simulink model "airTrackInelastic"  (R2021a)
settings: Solver=VariableStepAuto  StartTime=0.0  StopTime=30  FixedStep=0.02  MaxStep=0.01  RelTol=1e-6  EnableMultiTasking=on
PostLoadFcn:
  | disp('default settings')
  | 
  | % Default starting positions
  | x0_cart1 = -0.2
  | x0_cart2 = 0.8
  | x0_gate1 = -0.4
  | x0_gate2 = 0.4
  | 
  | % How much damping the carts feel
  | dampingCoef = 0.01 % N/(m/s)
  | 
  | % Max measurement noise for the gates
  | noise_max = 0.01 % seconds
  | 
  | % How many time steps to show in the history
  | nHistory = 4
  | 
  | % Based on the provided STLs
  | cart_length = 0.15
  | 
  | subsystems = find_system(gcs,'BlockType','SubSystem');
  | p = Simulink.Mask.get(subsystems{1});
  | p.Parameters(1).Value = '-0.8';
  | p.Parameters(2).Value = '0';
  | p.Parameters(3).Value = '-0.4';
  | p.Parameters(4).Value = '0.4';
  | p.Parameters(5).Value = '0';
  | p.Parameters(6).Value = '0';
undefined symbols (not defined in the file): Push, X, x, Y, Z
libraries: sm_lib x54, simulink x12, nesl_utility x11
(part 2 of 2)

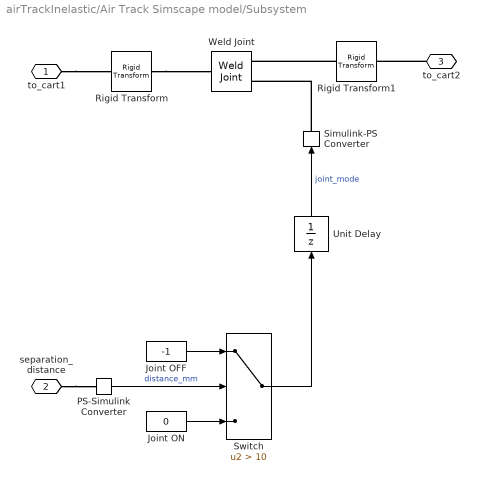
== system airTrackInelastic/Air Track Simscape model/Subsystem ==
  Joint OFF : Constant  Value=-1
  Joint ON : Constant  Value=0
  PS-Simulink Converter : nesl_utility/PS-Simulink Converter  PhysicalDomain=network_engine_domain  SubClassName=ps_output  LeftPortType=input  RightPortType=output  PseudoPeriodic=off  Frequencies=[]  Unit=mm  AffineConversion=off
      settings: SourceProductBaseCode=PW,SS
  Rigid Transform : sm_lib/Frames and Transforms/Rigid Transform  TranslationMethod=StandardAxis  TranslationStandardOffset=-0.0075  TranslationLengthUnit=m  TranslationStandardAxis=+X  TranslationCartesianOffset=[0 0 0]  TranslationROffset=0  TranslationROffsetUnits=m  TranslationZOffset=0  TranslationZOffsetUnits=m  TranslationThetaOffset=0  TranslationThetaOffsetUnits=deg  RotationMethod=None  RotationAngleUnits=deg  RotationStandardAxis=+Z  RotationAngle=0.0  RotationArbitraryAxis=[0 0 1]  FollAlignAxisA=+X  BaseAlignAxisA=+Y  FollAlignAxisB=+Y  BaseAlignAxisB=+Z  RotationSequenceAxes=FollowerAxes  RotationSequence=XYX  RotationSequenceAngles=[0 0 0]  RotationSequenceAnglesUnits=deg  RotationMatrix=[1 0 0; 0 1 0; 0 0 1]
  Rigid Transform1 : sm_lib/Frames and Transforms/Rigid Transform  TranslationMethod=StandardAxis  TranslationStandardOffset=0.0075  TranslationLengthUnit=m  TranslationStandardAxis=-X  TranslationCartesianOffset=[0 0 0]  TranslationROffset=0  TranslationROffsetUnits=m  TranslationZOffset=0  TranslationZOffsetUnits=m  TranslationThetaOffset=0  TranslationThetaOffsetUnits=deg  RotationMethod=None  RotationAngleUnits=deg  RotationStandardAxis=+Z  RotationAngle=0.0  RotationArbitraryAxis=[0 0 1]  FollAlignAxisA=+X  BaseAlignAxisA=+Y  FollAlignAxisB=+Y  BaseAlignAxisB=+Z  RotationSequenceAxes=FollowerAxes  RotationSequence=XYX  RotationSequenceAngles=[0 0 0]  RotationSequenceAnglesUnits=deg  RotationMatrix=[1 0 0; 0 1 0; 0 0 1]
  Simulink-PS Converter : nesl_utility/Simulink-PS Converter  PhysicalDomain=network_engine_domain  SubClassName=ps_input  LeftPortType=input  RightPortType=output  PseudoPeriodic=off  Frequencies=[]  NoiseDistribution=none  NoiseParameters=[]  Unit=1  AffineConversion=off  FilteringAndDerivatives=provide  SimscapeFilterOrder=1  InputFilterTimeConstant=0.001  UdotUserProvided=0
      settings: SourceProductBaseCode=PW,SS
  Switch : Switch  Criteria=u2 > Threshold  Threshold=10
  Unit Delay : UnitDelay  InitialCondition=-1  SampleTime=0.01  HasFrameUpgradeWarning=on
  Weld Joint : sm_lib/Joints/Weld Joint  JointMode=ProvidedByInput  SenseConstraintForce=off  SenseConstraintForceX=off  SenseConstraintForceY=off  SenseConstraintForceZ=off  SenseConstraintTorque=off  SenseConstraintTorqueX=off  SenseConstraintTorqueY=off  SenseConstraintTorqueZ=off  SenseTotalForce=off  SenseTotalForceX=off  SenseTotalForceY=off  SenseTotalForceZ=off  SenseTotalTorque=off  SenseTotalTorqueX=off  SenseTotalTorqueY=off  SenseTotalTorqueZ=off  CompositeWrenchDir=FollowerOnBase  CompositeWrenchFrame=BaseFrame
  to_cart1 : PMIOPort  Side=Left
  separation_distance : PMIOPort  Port=2  Side=Left
  to_cart2 : PMIOPort  Port=3  Side=Right
  wires:
  PS-Simulink Converter/1 -> Switch/2  "distance_mm"
  Joint OFF/1 -> Switch/1
  Joint ON/1 -> Switch/3
  Unit Delay/1 -> Simulink-PS Converter/1  "joint_mode"
  Switch/1 -> Unit Delay/1
  connections:
  to_cart2/RConn1 -- Rigid Transform1/RConn1
  Simulink-PS Converter/RConn1 -- Weld Joint/LConn2
  to_cart1/RConn1 -- Rigid Transform/LConn1
  separation_distance/RConn1 -- PS-Simulink Converter/LConn1
  Rigid Transform/RConn1 -- Weld Joint/RConn1
  Rigid Transform1/LConn1 -- Weld Joint/LConn1

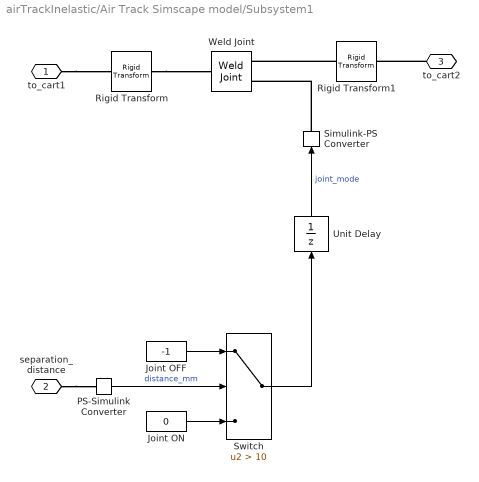
== system airTrackInelastic/Air Track Simscape model/Subsystem1 ==
  Joint OFF : Constant  Value=-1
  Joint ON : Constant  Value=0
  PS-Simulink Converter : nesl_utility/PS-Simulink Converter  PhysicalDomain=network_engine_domain  SubClassName=ps_output  LeftPortType=input  RightPortType=output  PseudoPeriodic=off  Frequencies=[]  Unit=mm  AffineConversion=off
      settings: SourceProductBaseCode=PW,SS
  Rigid Transform : sm_lib/Frames and Transforms/Rigid Transform  TranslationMethod=StandardAxis  TranslationStandardOffset=-0.0075  TranslationLengthUnit=m  TranslationStandardAxis=+X  TranslationCartesianOffset=[0 0 0]  TranslationROffset=0  TranslationROffsetUnits=m  TranslationZOffset=0  TranslationZOffsetUnits=m  TranslationThetaOffset=0  TranslationThetaOffsetUnits=deg  RotationMethod=None  RotationAngleUnits=deg  RotationStandardAxis=+Z  RotationAngle=0.0  RotationArbitraryAxis=[0 0 1]  FollAlignAxisA=+X  BaseAlignAxisA=+Y  FollAlignAxisB=+Y  BaseAlignAxisB=+Z  RotationSequenceAxes=FollowerAxes  RotationSequence=XYX  RotationSequenceAngles=[0 0 0]  RotationSequenceAnglesUnits=deg  RotationMatrix=[1 0 0; 0 1 0; 0 0 1]
  Rigid Transform1 : sm_lib/Frames and Transforms/Rigid Transform  TranslationMethod=StandardAxis  TranslationStandardOffset=0.0075  TranslationLengthUnit=m  TranslationStandardAxis=-X  TranslationCartesianOffset=[0 0 0]  TranslationROffset=0  TranslationROffsetUnits=m  TranslationZOffset=0  TranslationZOffsetUnits=m  TranslationThetaOffset=0  TranslationThetaOffsetUnits=deg  RotationMethod=None  RotationAngleUnits=deg  RotationStandardAxis=+Z  RotationAngle=0.0  RotationArbitraryAxis=[0 0 1]  FollAlignAxisA=+X  BaseAlignAxisA=+Y  FollAlignAxisB=+Y  BaseAlignAxisB=+Z  RotationSequenceAxes=FollowerAxes  RotationSequence=XYX  RotationSequenceAngles=[0 0 0]  RotationSequenceAnglesUnits=deg  RotationMatrix=[1 0 0; 0 1 0; 0 0 1]
  Simulink-PS Converter : nesl_utility/Simulink-PS Converter  PhysicalDomain=network_engine_domain  SubClassName=ps_input  LeftPortType=input  RightPortType=output  PseudoPeriodic=off  Frequencies=[]  NoiseDistribution=none  NoiseParameters=[]  Unit=1  AffineConversion=off  FilteringAndDerivatives=provide  SimscapeFilterOrder=1  InputFilterTimeConstant=0.001  UdotUserProvided=0
      settings: SourceProductBaseCode=PW,SS
  Switch : Switch  Criteria=u2 > Threshold  Threshold=10
  Unit Delay : UnitDelay  InitialCondition=-1  SampleTime=0.01  HasFrameUpgradeWarning=on
  Weld Joint : sm_lib/Joints/Weld Joint  JointMode=ProvidedByInput  SenseConstraintForce=off  SenseConstraintForceX=off  SenseConstraintForceY=off  SenseConstraintForceZ=off  SenseConstraintTorque=off  SenseConstraintTorqueX=off  SenseConstraintTorqueY=off  SenseConstraintTorqueZ=off  SenseTotalForce=off  SenseTotalForceX=off  SenseTotalForceY=off  SenseTotalForceZ=off  SenseTotalTorque=off  SenseTotalTorqueX=off  SenseTotalTorqueY=off  SenseTotalTorqueZ=off  CompositeWrenchDir=FollowerOnBase  CompositeWrenchFrame=BaseFrame
  to_cart1 : PMIOPort  Side=Left
  separation_distance : PMIOPort  Port=2  Side=Left
  to_cart2 : PMIOPort  Port=3  Side=Right
  wires:
  PS-Simulink Converter/1 -> Switch/2  "distance_mm"
  Joint OFF/1 -> Switch/1
  Joint ON/1 -> Switch/3
  Unit Delay/1 -> Simulink-PS Converter/1  "joint_mode"
  Switch/1 -> Unit Delay/1
  connections:
  to_cart2/RConn1 -- Rigid Transform1/RConn1
  Simulink-PS Converter/RConn1 -- Weld Joint/LConn2
  to_cart1/RConn1 -- Rigid Transform/LConn1
  separation_distance/RConn1 -- PS-Simulink Converter/LConn1
  Rigid Transform/RConn1 -- Weld Joint/RConn1
  Rigid Transform1/LConn1 -- Weld Joint/LConn1

== system airTrackInelastic/Air Track Simscape model/gate1 ==
  Constant : Constant  Value=x0_gate1
  Display : Display
  File Solid4 : sm_lib/Body Elements/File Solid  ExtGeomFileName=./stls/gate.stl  UnitType=Custom  ExtGeomFileUnits=mm  StepReaderType=HEX  ExportConvexHullGeometry=off  InertiaType=PointMass  Mass=180  MassUnits=g  CenterOfMass=[0 0 0]  CenterOfMassUnits=m  MomentsOfInertia=[1 1 1]  MomentsOfInertiaUnits=kg*m^2  ProductsOfInertia=[0 0 0]  ProductsOfInertiaUnits=kg*m^2  BasedOnType=Density  Density=1000  DensityUnits=kg/m^3  DoExposeReferenceFrame=on  SerializedFrames=<Frames><Frame><Id>Frame1</Id><Value><Name>F1</Name><Origin><Source>CenterOfMassFrame</Source><FeatureName></FeatureName></Origin><PrimaryAxis><DefinedDirection>+X</DefinedDirection><Source>ReferenceFrame</Source><SourceDirection>+Z</SourceDirection><FeatureName></FeatureName></PrimaryAxis><SecondaryAxis><DefinedDirection>+Y</DefinedDirection><Source>ReferenceFrame</Source><SourceDirection>+X</SourceDirection><FeatureName></FeatureName></SecondaryAxis></Value></Frame></Frames>  GraphicType=FromGeometry  MarkerShape=Sphere  MarkerSize=10  GraphicVisPropType=AdvancedVisualProperties  GraphicDiffuseColor="[0.8500    0.3250    0.0980]"  GraphicSpecularColor="[0.8    0.8   0.8 1]"  GraphicAmbientColor=[0.05 0.05 0.05 1]  GraphicEmissiveColor=[0.0 0.0 0.0 1.0]  GraphicShininess=50  GraphicOpacity=1.0
  Gate timing and history : Subsystem
  Rigid Transform : sm_lib/Frames and Transforms/Rigid Transform  TranslationMethod=Cartesian  TranslationStandardOffset=x0_cart2  TranslationLengthUnit=m  TranslationStandardAxis=+X  TranslationCartesianOffset=[-x0_gate1 0 0 ]  TranslationROffset=0  TranslationROffsetUnits=m  TranslationZOffset=0  TranslationZOffsetUnits=m  TranslationThetaOffset=0  TranslationThetaOffsetUnits=deg  RotationMethod=None  RotationAngleUnits=deg  RotationStandardAxis=+Z  RotationAngle=0.0  RotationArbitraryAxis=[0 0 1]  FollAlignAxisA=+X  BaseAlignAxisA=+Y  FollAlignAxisB=+Y  BaseAlignAxisB=+Z  RotationSequenceAxes=FollowerAxes  RotationSequence=XYX  RotationSequenceAngles=[0 0 0]  RotationSequenceAnglesUnits=deg  RotationMatrix=[1 0 0; 0 1 0; 0 0 1]
  File Solid3 : PMIOPort  Side=Right
  wires:
  Gate timing and history/1(Out1) -> Display/1
  Constant/1 -> Gate timing and history/1(gate_pos)
  connections:
  Rigid Transform/LConn1 -- File Solid3/RConn1
  File Solid4/RConn1 -- Rigid Transform/RConn1

== system airTrackInelastic/Air Track Simscape model/gate2 ==
  note: The cart has a mass of 180 grams and a length of 15cm
  Constant : Constant  Value=x0_gate2
  Display : Display
  File Solid4 : sm_lib/Body Elements/File Solid  ExtGeomFileName=./stls/gate.stl  UnitType=Custom  ExtGeomFileUnits=mm  StepReaderType=HEX  ExportConvexHullGeometry=off  InertiaType=PointMass  Mass=180  MassUnits=g  CenterOfMass=[0 0 0]  CenterOfMassUnits=m  MomentsOfInertia=[1 1 1]  MomentsOfInertiaUnits=kg*m^2  ProductsOfInertia=[0 0 0]  ProductsOfInertiaUnits=kg*m^2  BasedOnType=Density  Density=1000  DensityUnits=kg/m^3  DoExposeReferenceFrame=on  SerializedFrames=<Frames><Frame><Id>Frame1</Id><Value><Name>F1</Name><Origin><Source>CenterOfMassFrame</Source><FeatureName></FeatureName></Origin><PrimaryAxis><DefinedDirection>+X</DefinedDirection><Source>ReferenceFrame</Source><SourceDirection>+Z</SourceDirection><FeatureName></FeatureName></PrimaryAxis><SecondaryAxis><DefinedDirection>+Y</DefinedDirection><Source>ReferenceFrame</Source><SourceDirection>+X</SourceDirection><FeatureName></FeatureName></SecondaryAxis></Value></Frame></Frames>  GraphicType=FromGeometry  MarkerShape=Sphere  MarkerSize=10  GraphicVisPropType=AdvancedVisualProperties  GraphicDiffuseColor="[           0    0.4470    0.7410]"  GraphicSpecularColor="[0.8    0.8   0.8 1]"  GraphicAmbientColor=[0.05 0.05 0.05 1]  GraphicEmissiveColor=[0.0 0.0 0.0 1.0]  GraphicShininess=50  GraphicOpacity=1.0
  Gate timing and history : Subsystem
  Rigid Transform : sm_lib/Frames and Transforms/Rigid Transform  TranslationMethod=Cartesian  TranslationStandardOffset=x0_cart2  TranslationLengthUnit=m  TranslationStandardAxis=+X  TranslationCartesianOffset=[-x0_gate2 0 0]  TranslationROffset=0  TranslationROffsetUnits=m  TranslationZOffset=0  TranslationZOffsetUnits=m  TranslationThetaOffset=0  TranslationThetaOffsetUnits=deg  RotationMethod=None  RotationAngleUnits=deg  RotationStandardAxis=+Z  RotationAngle=0.0  RotationArbitraryAxis=[0 0 1]  FollAlignAxisA=+X  BaseAlignAxisA=+Y  FollAlignAxisB=+Y  BaseAlignAxisB=+Z  RotationSequenceAxes=FollowerAxes  RotationSequence=XYX  RotationSequenceAngles=[0 0 0]  RotationSequenceAnglesUnits=deg  RotationMatrix=[1 0 0; 0 1 0; 0 0 1]
  File Solid3 : PMIOPort  Side=Right
  wires:
  Constant/1 -> Gate timing and history/1(gate_pos)
  Gate timing and history/1(Out1) -> Display/1
  connections:
  File Solid4/RConn1 -- Rigid Transform/RConn1
  Rigid Transform/LConn1 -- File Solid3/RConn1

== system airTrackInelastic/Air Track Simscape model/stop1 ==
  File Solid2 : sm_lib/Body Elements/File Solid  ExtGeomFileName=./stls/stop.stl  UnitType=Custom  ExtGeomFileUnits=mm  StepReaderType=HEX  ExportConvexHullGeometry=off  InertiaType=PointMass  Mass=180  MassUnits=g  CenterOfMass=[0 0 0]  CenterOfMassUnits=m  MomentsOfInertia=[1 1 1]  MomentsOfInertiaUnits=kg*m^2  ProductsOfInertia=[0 0 0]  ProductsOfInertiaUnits=kg*m^2  BasedOnType=Density  Density=1000  DensityUnits=kg/m^3  DoExposeReferenceFrame=on  SerializedFrames=<Frames><Frame><Id>Frame1</Id><Value><Name>F1</Name><Origin><Source>CenterOfMassFrame</Source><FeatureName></FeatureName></Origin><PrimaryAxis><DefinedDirection>+X</DefinedDirection><Source>ReferenceFrame</Source><SourceDirection>+Z</SourceDirection><FeatureName></FeatureName></PrimaryAxis><SecondaryAxis><DefinedDirection>+Y</DefinedDirection><Source>ReferenceFrame</Source><SourceDirection>+X</SourceDirection><FeatureName></FeatureName></SecondaryAxis></Value></Frame></Frames>  GraphicType=FromGeometry  MarkerShape=Sphere  MarkerSize=10  GraphicVisPropType=AdvancedVisualProperties  GraphicDiffuseColor="[0.2   0.2    0.2]"  GraphicSpecularColor="[0.8    0.8   0.8 1]"  GraphicAmbientColor=[0.05 0.05 0.05 1]  GraphicEmissiveColor=[0.0 0.0 0.0 1.0]  GraphicShininess=50  GraphicOpacity=1.0
  Rigid Transform : sm_lib/Frames and Transforms/Rigid Transform  TranslationMethod=Cartesian  TranslationStandardOffset=0  TranslationLengthUnit=m  TranslationStandardAxis=+X  TranslationCartesianOffset=[0 0 0]  TranslationROffset=0  TranslationROffsetUnits=m  TranslationZOffset=0  TranslationZOffsetUnits=m  TranslationThetaOffset=0  TranslationThetaOffsetUnits=deg  RotationMethod=None  RotationAngleUnits=deg  RotationStandardAxis=+Z  RotationAngle=0.0  RotationArbitraryAxis=[0 0 1]  FollAlignAxisA=+X  BaseAlignAxisA=+Y  FollAlignAxisB=+Y  BaseAlignAxisB=+Z  RotationSequenceAxes=FollowerAxes  RotationSequence=XYX  RotationSequenceAngles=[0 0 0]  RotationSequenceAnglesUnits=deg  RotationMatrix=[1 0 0; 0 1 0; 0 0 1]
  Rigid Transform1 : sm_lib/Frames and Transforms/Rigid Transform  TranslationMethod=Cartesian  TranslationStandardOffset=1  TranslationLengthUnit=m  TranslationStandardAxis=+X  TranslationCartesianOffset=[1-0.012 -0.225 0]  TranslationROffset=0  TranslationROffsetUnits=m  TranslationZOffset=0  TranslationZOffsetUnits=m  TranslationThetaOffset=0  TranslationThetaOffsetUnits=deg  RotationMethod=None  RotationAngleUnits=deg  RotationStandardAxis=+Z  RotationAngle=0.0  RotationArbitraryAxis=[0 0 1]  FollAlignAxisA=+X  BaseAlignAxisA=+Y  FollAlignAxisB=+Y  BaseAlignAxisB=+Z  RotationSequenceAxes=FollowerAxes  RotationSequence=XYX  RotationSequenceAngles=[0 0 0]  RotationSequenceAnglesUnits=deg  RotationMatrix=[1 0 0; 0 1 0; 0 0 1]
  contact_ball1 : sm_lib/Body Elements/Spherical Solid  GraphicAmbientColor=[0.15 0.15 0.15 1.0]  BasedOnType=Density  CenterOfMass=[0 0 0]  CenterOfMassUnits=m  GraphicDiffuseColor="[ 0.9290    0.6940    0.1250]"  Density=1000  DensityUnits=kg/m^3  DoExposeReferenceFrame=on  GraphicEmissiveColor=[0.0 0.0 0.0 1.0]  ExportEntireGeometry=on  SerializedExposedGeometries=<ExposedGeometries><ExposedGeometry><RawGeometryId>entire</RawGeometryId><ExposedGeometryId>G</ExposedGeometryId></ExposedGeometry></ExposedGeometries>  SerializedFrames=<Frames/>  MarkerShape=Sphere  MarkerSize=10  GraphicType=FromGeometry  InertiaType=CalculateFromGeometry  Mass=1  MassUnits=kg  MomentsOfInertia=[1 1 1]  MomentsOfInertiaUnits=kg*m^2  GraphicOpacity=1.0  ProductsOfInertia=[0 0 0]  ProductsOfInertiaUnits=kg*m^2  GraphicShininess=75  GraphicSpecularColor=[0.5 0.5 0.5 1.0]  SphereRadius=0.0075  SphereRadiusUnits=m  GraphicVisPropType=SimpleVisualProperties
  File Solid1 : PMIOPort  Side=Left
  File Solid3 : PMIOPort  Port=2  Side=Right
  contact : PMIOPort  Port=3  Side=Left
  connections:
  Rigid Transform/LConn1 -- File Solid3/RConn1
  File Solid1/RConn1 -- Rigid Transform1/RConn1 -- Rigid Transform/RConn1 -- File Solid2/RConn1
  contact_ball1/RConn1 -- Rigid Transform1/LConn1
  contact/RConn1 -- contact_ball1/LConn1

== system airTrackInelastic/Air Track Simscape model/stop2 ==
  File Solid2 : sm_lib/Body Elements/File Solid  ExtGeomFileName=./stls/stop.stl  UnitType=Custom  ExtGeomFileUnits=mm  StepReaderType=HEX  ExportConvexHullGeometry=off  InertiaType=PointMass  Mass=180  MassUnits=g  CenterOfMass=[0 0 0]  CenterOfMassUnits=m  MomentsOfInertia=[1 1 1]  MomentsOfInertiaUnits=kg*m^2  ProductsOfInertia=[0 0 0]  ProductsOfInertiaUnits=kg*m^2  BasedOnType=Density  Density=1000  DensityUnits=kg/m^3  DoExposeReferenceFrame=on  SerializedFrames=<Frames><Frame><Id>Frame1</Id><Value><Name>F1</Name><Origin><Source>CenterOfMassFrame</Source><FeatureName></FeatureName></Origin><PrimaryAxis><DefinedDirection>+Z</DefinedDirection><Source>ReferenceFrame</Source><SourceDirection>+Z</SourceDirection><FeatureName></FeatureName></PrimaryAxis><SecondaryAxis><DefinedDirection>+X</DefinedDirection><Source>ReferenceFrame</Source><SourceDirection>+X</SourceDirection><FeatureName></FeatureName></SecondaryAxis></Value></Frame></Frames>  GraphicType=FromGeometry  MarkerShape=Sphere  MarkerSize=10  GraphicVisPropType=AdvancedVisualProperties  GraphicDiffuseColor="[0.2   0.2    0.2]"  GraphicSpecularColor="[0.8    0.8   0.8 1]"  GraphicAmbientColor=[0.05 0.05 0.05 1]  GraphicEmissiveColor=[0.0 0.0 0.0 1.0]  GraphicShininess=50  GraphicOpacity=1.0
  Rigid Transform : sm_lib/Frames and Transforms/Rigid Transform  TranslationMethod=StandardAxis  TranslationStandardOffset=1.985  TranslationLengthUnit=m  TranslationStandardAxis=+X  TranslationCartesianOffset=[0 0 0]  TranslationROffset=0  TranslationROffsetUnits=m  TranslationZOffset=0  TranslationZOffsetUnits=m  TranslationThetaOffset=0  TranslationThetaOffsetUnits=deg  RotationMethod=None  RotationAngleUnits=deg  RotationStandardAxis=+Z  RotationAngle=0.0  RotationArbitraryAxis=[0 0 1]  FollAlignAxisA=+X  BaseAlignAxisA=+Y  FollAlignAxisB=+Y  BaseAlignAxisB=+Z  RotationSequenceAxes=FollowerAxes  RotationSequence=XYX  RotationSequenceAngles=[0 0 0]  RotationSequenceAnglesUnits=deg  RotationMatrix=[1 0 0; 0 1 0; 0 0 1]
  Rigid Transform1 : sm_lib/Frames and Transforms/Rigid Transform  TranslationMethod=Cartesian  TranslationStandardOffset=1  TranslationLengthUnit=m  TranslationStandardAxis=+X  TranslationCartesianOffset=[1-0.003 -0.225 0]  TranslationROffset=0  TranslationROffsetUnits=m  TranslationZOffset=0  TranslationZOffsetUnits=m  TranslationThetaOffset=0  TranslationThetaOffsetUnits=deg  RotationMethod=None  RotationAngleUnits=deg  RotationStandardAxis=+Z  RotationAngle=0.0  RotationArbitraryAxis=[0 0 1]  FollAlignAxisA=+X  BaseAlignAxisA=+Y  FollAlignAxisB=+Y  BaseAlignAxisB=+Z  RotationSequenceAxes=FollowerAxes  RotationSequence=XYX  RotationSequenceAngles=[0 0 0]  RotationSequenceAnglesUnits=deg  RotationMatrix=[1 0 0; 0 1 0; 0 0 1]
  contact_ball1 : sm_lib/Body Elements/Spherical Solid  GraphicAmbientColor=[0.15 0.15 0.15 1.0]  BasedOnType=Density  CenterOfMass=[0 0 0]  CenterOfMassUnits=m  GraphicDiffuseColor="[ 0.9290    0.6940    0.1250]"  Density=1000  DensityUnits=kg/m^3  DoExposeReferenceFrame=on  GraphicEmissiveColor=[0.0 0.0 0.0 1.0]  ExportEntireGeometry=on  SerializedExposedGeometries=<ExposedGeometries><ExposedGeometry><RawGeometryId>entire</RawGeometryId><ExposedGeometryId>G</ExposedGeometryId></ExposedGeometry></ExposedGeometries>  SerializedFrames=<Frames/>  MarkerShape=Sphere  MarkerSize=10  GraphicType=FromGeometry  InertiaType=CalculateFromGeometry  Mass=1  MassUnits=kg  MomentsOfInertia=[1 1 1]  MomentsOfInertiaUnits=kg*m^2  GraphicOpacity=1.0  ProductsOfInertia=[0 0 0]  ProductsOfInertiaUnits=kg*m^2  GraphicShininess=75  GraphicSpecularColor=[0.5 0.5 0.5 1.0]  SphereRadius=0.0075  SphereRadiusUnits=m  GraphicVisPropType=SimpleVisualProperties
  File Solid1 : PMIOPort  Side=Left
  File Solid3 : PMIOPort  Port=2  Side=Right
  contact : PMIOPort  Port=3  Side=Left
  connections:
  contact_ball1/RConn1 -- Rigid Transform1/LConn1
  Rigid Transform/LConn1 -- File Solid3/RConn1
  Rigid Transform1/RConn1 -- File Solid2/RConn1 -- Rigid Transform/RConn1 -- File Solid1/RConn1
  contact/RConn1 -- contact_ball1/LConn1

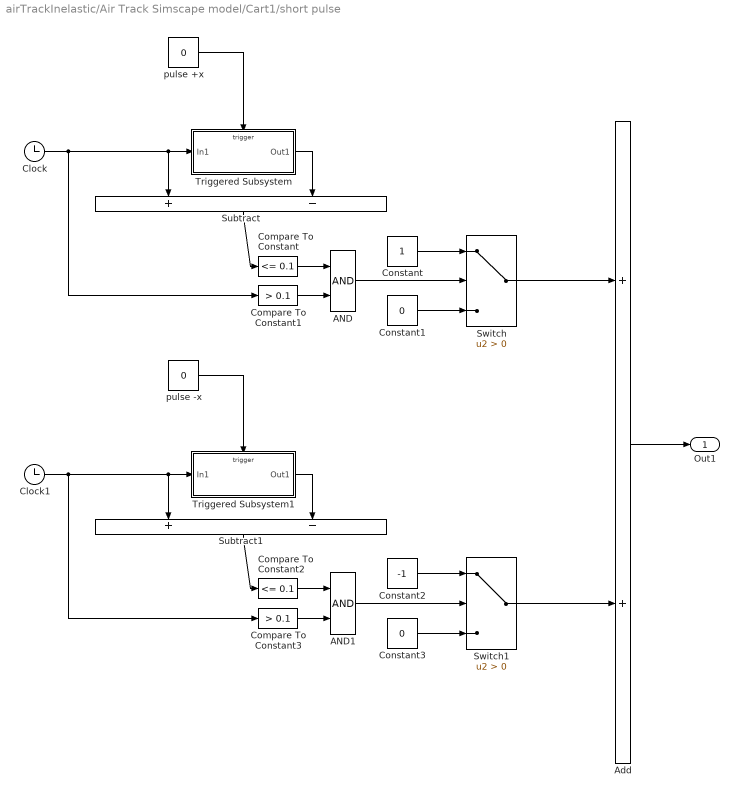
== system airTrackInelastic/Air Track Simscape model/Cart1/short pulse ==
  AND : Logic  IconShape=distinctive  AllPortsSameDT=off  OutDataTypeStr=boolean
  AND1 : Logic  IconShape=distinctive  AllPortsSameDT=off  OutDataTypeStr=boolean
  Add : Sum
  Clock : Clock
  Clock1 : Clock
  Compare To Constant : simulink/Logic and Bit Operations/Compare To Constant  relop=<=  const=0.1  OutDataTypeStr=boolean
  Compare To Constant1 : simulink/Logic and Bit Operations/Compare To Constant  relop=>  const=0.1  OutDataTypeStr=boolean
  Compare To Constant2 : simulink/Logic and Bit Operations/Compare To Constant  relop=<=  const=0.1  OutDataTypeStr=boolean
  Compare To Constant3 : simulink/Logic and Bit Operations/Compare To Constant  relop=>  const=0.1  OutDataTypeStr=boolean
  Constant : Constant
  Constant1 : Constant  Value=0
  Constant2 : Constant  Value=-1
  Constant3 : Constant  Value=0
  Subtract : Sum  Inputs=+-
  Subtract1 : Sum  Inputs=+-
  Switch : Switch  Criteria=u2 > Threshold
  Switch1 : Switch  Criteria=u2 > Threshold
  Triggered Subsystem : Subsystem  TreatAsAtomicUnit=on
  Triggered Subsystem1 : Subsystem  TreatAsAtomicUnit=on
  pulse +x : Constant  Value=0
  pulse -x : Constant  Value=0
  Out1 : Outport
  wires:
  pulse +x/1 -> Triggered Subsystem/Trigger
  Triggered Subsystem/1(Out1) -> Subtract/2
  Constant/1 -> Switch/1
  Subtract/1 -> Compare To Constant/1
  Constant1/1 -> Switch/3
  AND/1 -> Switch/2
  Compare To Constant/1 -> AND/1
  Clock/1 -> Compare To Constant1/1, Triggered Subsystem/1(In1), Subtract/1
  Compare To Constant1/1 -> AND/2
  Switch/1 -> Add/1
  Add/1 -> Out1/1
  Compare To Constant3/1 -> AND1/2
  Switch1/1 -> Add/2
  pulse -x/1 -> Triggered Subsystem1/Trigger
  Clock1/1 -> Compare To Constant3/1, Triggered Subsystem1/1(In1), Subtract1/1
  Constant3/1 -> Switch1/3
  Compare To Constant2/1 -> AND1/1
  Subtract1/1 -> Compare To Constant2/1
  Constant2/1 -> Switch1/1
  AND1/1 -> Switch1/2
  Triggered Subsystem1/1(Out1) -> Subtract1/2

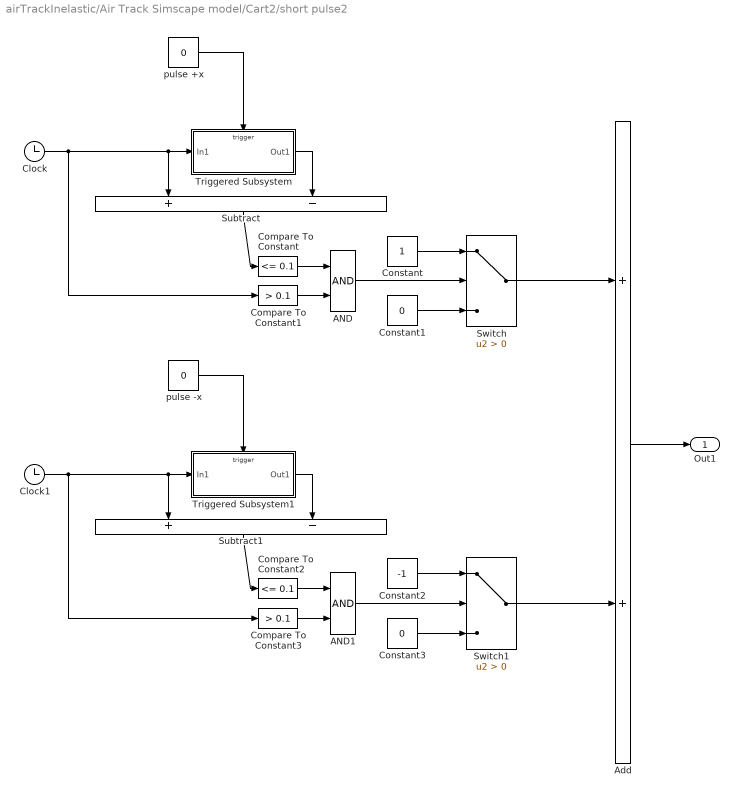
== system airTrackInelastic/Air Track Simscape model/Cart2/short pulse2 ==
  AND : Logic  IconShape=distinctive  AllPortsSameDT=off  OutDataTypeStr=boolean
  AND1 : Logic  IconShape=distinctive  AllPortsSameDT=off  OutDataTypeStr=boolean
  Add : Sum
  Clock : Clock
  Clock1 : Clock
  Compare To Constant : simulink/Logic and Bit Operations/Compare To Constant  relop=<=  const=0.1  OutDataTypeStr=boolean
  Compare To Constant1 : simulink/Logic and Bit Operations/Compare To Constant  relop=>  const=0.1  OutDataTypeStr=boolean
  Compare To Constant2 : simulink/Logic and Bit Operations/Compare To Constant  relop=<=  const=0.1  OutDataTypeStr=boolean
  Compare To Constant3 : simulink/Logic and Bit Operations/Compare To Constant  relop=>  const=0.1  OutDataTypeStr=boolean
  Constant : Constant
  Constant1 : Constant  Value=0
  Constant2 : Constant  Value=-1
  Constant3 : Constant  Value=0
  Subtract : Sum  Inputs=+-
  Subtract1 : Sum  Inputs=+-
  Switch : Switch  Criteria=u2 > Threshold
  Switch1 : Switch  Criteria=u2 > Threshold
  Triggered Subsystem : Subsystem  TreatAsAtomicUnit=on
  Triggered Subsystem1 : Subsystem  TreatAsAtomicUnit=on
  pulse +x : Constant  Value=0
  pulse -x : Constant  Value=0
  Out1 : Outport
  wires:
  pulse +x/1 -> Triggered Subsystem/Trigger
  Triggered Subsystem/1(Out1) -> Subtract/2
  Constant/1 -> Switch/1
  Subtract/1 -> Compare To Constant/1
  Constant1/1 -> Switch/3
  AND/1 -> Switch/2
  Compare To Constant/1 -> AND/1
  Clock/1 -> Compare To Constant1/1, Triggered Subsystem/1(In1), Subtract/1
  Compare To Constant1/1 -> AND/2
  Switch/1 -> Add/1
  Add/1 -> Out1/1
  Compare To Constant3/1 -> AND1/2
  Switch1/1 -> Add/2
  pulse -x/1 -> Triggered Subsystem1/Trigger
  Clock1/1 -> Compare To Constant3/1, Triggered Subsystem1/1(In1), Subtract1/1
  Constant3/1 -> Switch1/3
  Compare To Constant2/1 -> AND1/1
  Subtract1/1 -> Compare To Constant2/1
  Constant2/1 -> Switch1/1
  AND1/1 -> Switch1/2
  Triggered Subsystem1/1(Out1) -> Subtract1/2

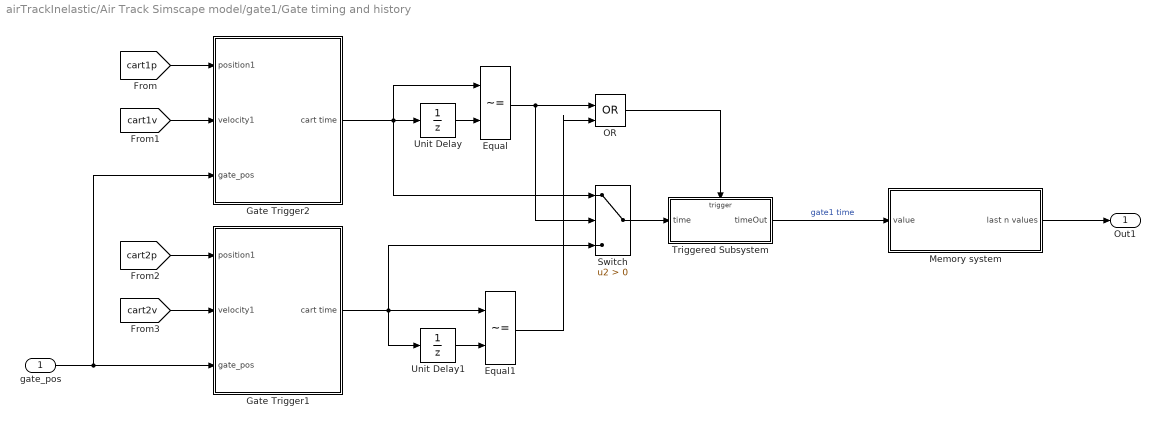
== system airTrackInelastic/Air Track Simscape model/gate1/Gate timing and history ==
  gate_pos : Inport
  Equal : RelationalOperator  Operator=~=  OutDataTypeStr=boolean  RndMeth=Simplest
  Equal1 : RelationalOperator  Operator=~=  OutDataTypeStr=boolean  RndMeth=Simplest
  Gate Trigger1 : Subsystem
  Gate Trigger2 : Subsystem
  Memory system : Subsystem
  OR : Logic  Operator=OR  IconShape=distinctive  AllPortsSameDT=off  OutDataTypeStr=boolean
  Switch : Switch  Criteria=u2 > Threshold
  Triggered Subsystem : Subsystem  TreatAsAtomicUnit=on
  Unit Delay : UnitDelay  SampleTime=-1  HasFrameUpgradeWarning=on
  Unit Delay1 : UnitDelay  SampleTime=-1  HasFrameUpgradeWarning=on
  Out1 : Outport
  wires:
  Gate Trigger1/1(cart time) -> Switch/3, Equal1/1, Unit Delay1/1
  gate_pos/1 -> Gate Trigger2/3(gate_pos), Gate Trigger1/3(gate_pos)
  OR/1 -> Triggered Subsystem/Trigger
  [cart2p] -> Gate Trigger1/1(position1)
  Equal/1 -> Switch/2, OR/1
  [cart1v] -> Gate Trigger2/2(velocity1)
  Triggered Subsystem/1(timeOut) -> Memory system/1(value)  "gate1 time"
  [cart2v] -> Gate Trigger1/2(velocity1)
  Unit Delay/1 -> Equal/2
  Gate Trigger2/1(cart time) -> Switch/1, Equal/1, Unit Delay/1
  Equal1/1 -> OR/2
  Unit Delay1/1 -> Equal1/2
  [cart1p] -> Gate Trigger2/1(position1)
  Switch/1 -> Triggered Subsystem/1(time)
  Memory system/1(last n values) -> Out1/1

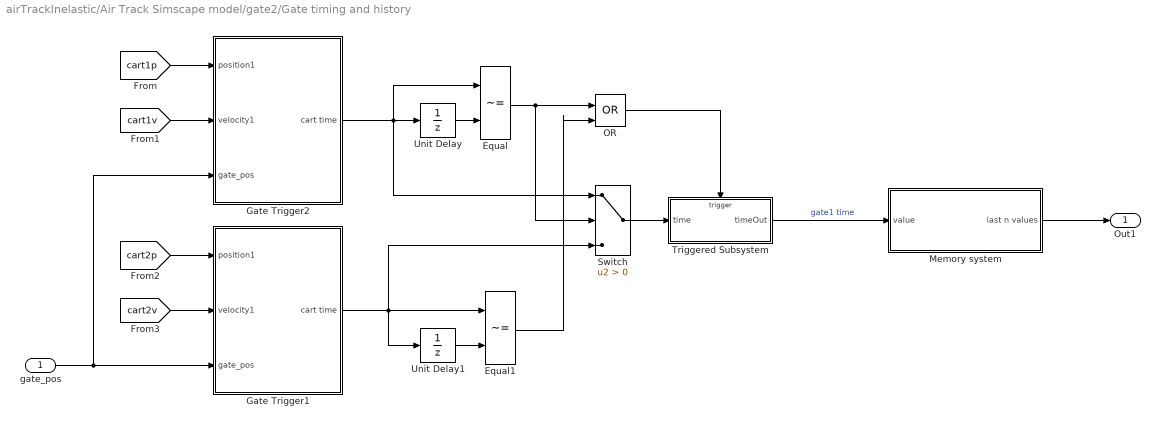
== system airTrackInelastic/Air Track Simscape model/gate2/Gate timing and history ==
  gate_pos : Inport
  Equal : RelationalOperator  Operator=~=  OutDataTypeStr=boolean  RndMeth=Simplest
  Equal1 : RelationalOperator  Operator=~=  OutDataTypeStr=boolean  RndMeth=Simplest
  Gate Trigger1 : Subsystem
  Gate Trigger2 : Subsystem
  Memory system : Subsystem
  OR : Logic  Operator=OR  IconShape=distinctive  AllPortsSameDT=off  OutDataTypeStr=boolean
  Switch : Switch  Criteria=u2 > Threshold
  Triggered Subsystem : Subsystem  TreatAsAtomicUnit=on
  Unit Delay : UnitDelay  SampleTime=-1  HasFrameUpgradeWarning=on
  Unit Delay1 : UnitDelay  SampleTime=-1  HasFrameUpgradeWarning=on
  Out1 : Outport
  wires:
  Gate Trigger1/1(cart time) -> Switch/3, Equal1/1, Unit Delay1/1
  gate_pos/1 -> Gate Trigger2/3(gate_pos), Gate Trigger1/3(gate_pos)
  OR/1 -> Triggered Subsystem/Trigger
  [cart2p] -> Gate Trigger1/1(position1)
  Equal/1 -> Switch/2, OR/1
  [cart1v] -> Gate Trigger2/2(velocity1)
  Triggered Subsystem/1(timeOut) -> Memory system/1(value)  "gate1 time"
  [cart2v] -> Gate Trigger1/2(velocity1)
  Unit Delay/1 -> Equal/2
  Gate Trigger2/1(cart time) -> Switch/1, Equal/1, Unit Delay/1
  Equal1/1 -> OR/2
  Unit Delay1/1 -> Equal1/2
  [cart1p] -> Gate Trigger2/1(position1)
  Switch/1 -> Triggered Subsystem/1(time)
  Memory system/1(last n values) -> Out1/1

== system airTrackInelastic/Air Track Simscape model/Cart1/short pulse/Triggered Subsystem ==
  In1 : Inport
  Trigger : TriggerPort  VariantControl=Variant
  Out1 : Outport
  wires:
  In1/1 -> Out1/1

== system airTrackInelastic/Air Track Simscape model/Cart1/short pulse/Triggered Subsystem1 ==
  In1 : Inport
  Trigger : TriggerPort  VariantControl=Variant
  Out1 : Outport
  wires:
  In1/1 -> Out1/1

== system airTrackInelastic/Air Track Simscape model/Cart2/short pulse2/Triggered Subsystem ==
  In1 : Inport
  Trigger : TriggerPort  VariantControl=Variant
  Out1 : Outport
  wires:
  In1/1 -> Out1/1

== system airTrackInelastic/Air Track Simscape model/Cart2/short pulse2/Triggered Subsystem1 ==
  In1 : Inport
  Trigger : TriggerPort  VariantControl=Variant
  Out1 : Outport
  wires:
  In1/1 -> Out1/1

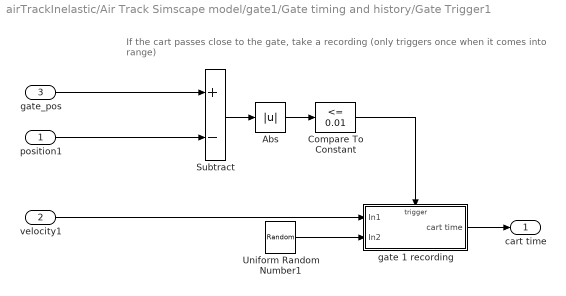
== system airTrackInelastic/Air Track Simscape model/gate1/Gate timing and history/Gate Trigger1 ==
  note: If the cart passes close to the gate, take a recording
      | (only triggers once when it comes into range)
  position1 : Inport
  velocity1 : Inport  Port=2
  gate_pos : Inport  Port=3
  Abs : Abs
  Compare To Constant : simulink/Logic and Bit Operations/Compare To Constant  relop=<=  const=0.01  OutDataTypeStr=boolean
  Subtract : Sum  Inputs=+-
  Uniform Random Number1 : UniformRandomNumber  Minimum=-noise_max/2  Maximum=noise_max/2  SampleTime=0.1
  gate 1 recording : Subsystem  TreatAsAtomicUnit=on
  cart time : Outport
  wires:
  position1/1 -> Subtract/2
  velocity1/1 -> gate 1 recording/1(In1)
  gate 1 recording/1(cart time) -> cart time/1
  Abs/1 -> Compare To Constant/1
  Subtract/1 -> Abs/1
  Compare To Constant/1 -> gate 1 recording/Trigger
  Uniform Random Number1/1 -> gate 1 recording/2(In2)
  gate_pos/1 -> Subtract/1

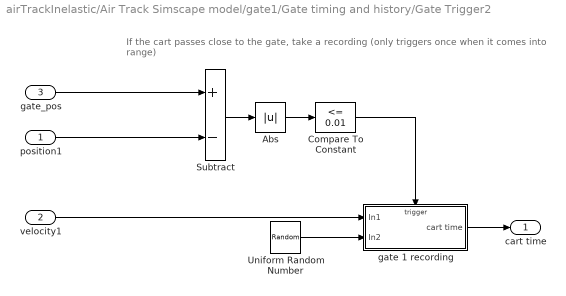
== system airTrackInelastic/Air Track Simscape model/gate1/Gate timing and history/Gate Trigger2 ==
  note: If the cart passes close to the gate, take a recording
      | (only triggers once when it comes into range)
  position1 : Inport
  velocity1 : Inport  Port=2
  gate_pos : Inport  Port=3
  Abs : Abs
  Compare To Constant : simulink/Logic and Bit Operations/Compare To Constant  relop=<=  const=0.01  OutDataTypeStr=boolean
  Subtract : Sum  Inputs=+-
  Uniform Random Number : UniformRandomNumber  Minimum=-noise_max/2  Maximum=noise_max/2  SampleTime=0.1
  gate 1 recording : Subsystem  TreatAsAtomicUnit=on
  cart time : Outport
  wires:
  position1/1 -> Subtract/2
  velocity1/1 -> gate 1 recording/1(In1)
  gate 1 recording/1(cart time) -> cart time/1
  Abs/1 -> Compare To Constant/1
  Subtract/1 -> Abs/1
  Compare To Constant/1 -> gate 1 recording/Trigger
  Uniform Random Number/1 -> gate 1 recording/2(In2)
  gate_pos/1 -> Subtract/1

== system airTrackInelastic/Air Track Simscape model/gate1/Gate timing and history/Memory system ==
  value : Inport
  Assignment : Assignment  DiagnosticForDimensions=Warning  IndexOptions=Index vector (dialog)  Indices=1  OutputSizes=1
  Equal : RelationalOperator  Operator=~=  OutDataTypeStr=boolean  RndMeth=Simplest
  Triggered Subsystem : Subsystem  TreatAsAtomicUnit=on
  Unit Delay : UnitDelay  InitialCondition=zeros(nHistory,1)  SampleTime=-1  HasFrameUpgradeWarning=on
  Unit Delay1 : UnitDelay  SampleTime=-1  HasFrameUpgradeWarning=on
  last n values : Outport
  wires:
  Unit Delay/1 -> Triggered Subsystem/1(In1)
  Assignment/1 -> Unit Delay/1, last n values/1
  value/1 -> Equal/1, Unit Delay1/1, Assignment/2
  Triggered Subsystem/1(Out1) -> Assignment/1
  Equal/1 -> Triggered Subsystem/Trigger
  Unit Delay1/1 -> Equal/2

== system airTrackInelastic/Air Track Simscape model/gate1/Gate timing and history/Triggered Subsystem ==
  time : Inport
  Trigger : TriggerPort  VariantControl=Variant
  timeOut : Outport
  wires:
  time/1 -> timeOut/1

== system airTrackInelastic/Air Track Simscape model/gate2/Gate timing and history/Gate Trigger1 ==
  note: If the cart passes close to the gate, take a recording
      | (only triggers once when it comes into range)
  position1 : Inport
  velocity1 : Inport  Port=2
  gate_pos : Inport  Port=3
  Abs : Abs
  Compare To Constant : simulink/Logic and Bit Operations/Compare To Constant  relop=<=  const=0.01  OutDataTypeStr=boolean
  Subtract : Sum  Inputs=+-
  Uniform Random Number1 : UniformRandomNumber  Minimum=-noise_max/2  Maximum=noise_max/2  SampleTime=0.1
  gate 1 recording : Subsystem  TreatAsAtomicUnit=on
  cart time : Outport
  wires:
  position1/1 -> Subtract/2
  velocity1/1 -> gate 1 recording/1(In1)
  gate 1 recording/1(cart time) -> cart time/1
  Abs/1 -> Compare To Constant/1
  Subtract/1 -> Abs/1
  Compare To Constant/1 -> gate 1 recording/Trigger
  Uniform Random Number1/1 -> gate 1 recording/2(In2)
  gate_pos/1 -> Subtract/1

== system airTrackInelastic/Air Track Simscape model/gate2/Gate timing and history/Gate Trigger2 ==
  note: If the cart passes close to the gate, take a recording
      | (only triggers once when it comes into range)
  position1 : Inport
  velocity1 : Inport  Port=2
  gate_pos : Inport  Port=3
  Abs : Abs
  Compare To Constant : simulink/Logic and Bit Operations/Compare To Constant  relop=<=  const=0.01  OutDataTypeStr=boolean
  Subtract : Sum  Inputs=+-
  Uniform Random Number1 : UniformRandomNumber  Minimum=-noise_max/2  Maximum=noise_max/2  SampleTime=0.1
  gate 1 recording : Subsystem  TreatAsAtomicUnit=on
  cart time : Outport
  wires:
  position1/1 -> Subtract/2
  velocity1/1 -> gate 1 recording/1(In1)
  gate 1 recording/1(cart time) -> cart time/1
  Abs/1 -> Compare To Constant/1
  Subtract/1 -> Abs/1
  Compare To Constant/1 -> gate 1 recording/Trigger
  Uniform Random Number1/1 -> gate 1 recording/2(In2)
  gate_pos/1 -> Subtract/1

== system airTrackInelastic/Air Track Simscape model/gate2/Gate timing and history/Memory system ==
  value : Inport
  Assignment : Assignment  DiagnosticForDimensions=Warning  IndexOptions=Index vector (dialog)  Indices=1  OutputSizes=1
  Equal : RelationalOperator  Operator=~=  OutDataTypeStr=boolean  RndMeth=Simplest
  Triggered Subsystem : Subsystem  TreatAsAtomicUnit=on
  Unit Delay : UnitDelay  InitialCondition=zeros(nHistory,1)  SampleTime=-1  HasFrameUpgradeWarning=on
  Unit Delay1 : UnitDelay  SampleTime=-1  HasFrameUpgradeWarning=on
  last n values : Outport
  wires:
  Unit Delay/1 -> Triggered Subsystem/1(In1)
  Assignment/1 -> Unit Delay/1, last n values/1
  value/1 -> Equal/1, Unit Delay1/1, Assignment/2
  Triggered Subsystem/1(Out1) -> Assignment/1
  Equal/1 -> Triggered Subsystem/Trigger
  Unit Delay1/1 -> Equal/2

== system airTrackInelastic/Air Track Simscape model/gate2/Gate timing and history/Triggered Subsystem ==
  time : Inport
  Trigger : TriggerPort  VariantControl=Variant
  timeOut : Outport
  wires:
  time/1 -> timeOut/1

== system airTrackInelastic/Air Track Simscape model/gate1/Gate timing and history/Gate Trigger1/gate 1 recording ==
  In1 : Inport
  In2 : Inport  Port=2
  Trigger : TriggerPort  VariantControl=Variant
  Abs : Abs
  Divide : Product  Inputs=*/
  Sum : Sum  Inputs=|++
  cart length (meters) : Constant  Value=cart_length
  cart time : Outport
  wires:
  In2/1 -> Sum/2
  Sum/1 -> cart time/1
  Abs/1 -> Sum/1
  Divide/1 -> Abs/1
  In1/1 -> Divide/2
  cart length (meters)/1 -> Divide/1

== system airTrackInelastic/Air Track Simscape model/gate1/Gate timing and history/Gate Trigger2/gate 1 recording ==
  In1 : Inport
  In2 : Inport  Port=2
  Trigger : TriggerPort  VariantControl=Variant
  Abs : Abs
  Divide : Product  Inputs=*/
  Sum : Sum  Inputs=|++
  cart length (meters) : Constant  Value=cart_length
  cart time : Outport
  wires:
  In2/1 -> Sum/2
  Sum/1 -> cart time/1
  Abs/1 -> Sum/1
  Divide/1 -> Abs/1
  In1/1 -> Divide/2
  cart length (meters)/1 -> Divide/1

== system airTrackInelastic/Air Track Simscape model/gate1/Gate timing and history/Memory system/Triggered Subsystem ==
  In1 : Inport
  Trigger : TriggerPort  VariantControl=Variant
  For Iterator Subsystem : Subsystem  TreatAsAtomicUnit=on
  Out1 : Outport
  wires:
  In1/1 -> For Iterator Subsystem/1(In1)
  For Iterator Subsystem/1(Out1) -> Out1/1

== system airTrackInelastic/Air Track Simscape model/gate2/Gate timing and history/Gate Trigger1/gate 1 recording ==
  In1 : Inport
  In2 : Inport  Port=2
  Trigger : TriggerPort  VariantControl=Variant
  Abs : Abs
  Divide : Product  Inputs=*/
  Sum : Sum  Inputs=|++
  cart length (meters) : Constant  Value=cart_length
  cart time : Outport
  wires:
  In2/1 -> Sum/2
  Sum/1 -> cart time/1
  Abs/1 -> Sum/1
  Divide/1 -> Abs/1
  In1/1 -> Divide/2
  cart length (meters)/1 -> Divide/1

== system airTrackInelastic/Air Track Simscape model/gate2/Gate timing and history/Gate Trigger2/gate 1 recording ==
  In1 : Inport
  In2 : Inport  Port=2
  Trigger : TriggerPort  VariantControl=Variant
  Abs : Abs
  Divide : Product  Inputs=*/
  Sum : Sum  Inputs=|++
  cart length (meters) : Constant  Value=cart_length
  cart time : Outport
  wires:
  In2/1 -> Sum/2
  Sum/1 -> cart time/1
  Abs/1 -> Sum/1
  Divide/1 -> Abs/1
  In1/1 -> Divide/2
  cart length (meters)/1 -> Divide/1

== system airTrackInelastic/Air Track Simscape model/gate2/Gate timing and history/Memory system/Triggered Subsystem ==
  In1 : Inport
  Trigger : TriggerPort  VariantControl=Variant
  For Iterator Subsystem : Subsystem  TreatAsAtomicUnit=on
  Out1 : Outport
  wires:
  In1/1 -> For Iterator Subsystem/1(In1)
  For Iterator Subsystem/1(Out1) -> Out1/1

== system airTrackInelastic/Air Track Simscape model/gate1/Gate timing and history/Memory system/Triggered Subsystem/For Iterator Subsystem ==
  In1 : Inport
  Assignment : Assignment  DiagnosticForDimensions=Warning  IndexOptions=Index vector (port)  Indices=1  OutputSizes=1
  Bias : Bias  Bias=1
  For Iterator : ForIterator  IterationLimit=nHistory-1
  Selector : Selector  InputPortWidth=nHistory  IndexOptions=Index vector (port)  Indices=[1 3]  OutputSizes=1
  Out1 : Outport
  wires:
  For Iterator/1 -> Bias/1, Selector/2
  Assignment/1 -> Out1/1
  In1/1 -> Assignment/1, Selector/1
  Bias/1 -> Assignment/3
  Selector/1 -> Assignment/2

== system airTrackInelastic/Air Track Simscape model/gate2/Gate timing and history/Memory system/Triggered Subsystem/For Iterator Subsystem ==
  In1 : Inport
  Assignment : Assignment  DiagnosticForDimensions=Warning  IndexOptions=Index vector (port)  Indices=1  OutputSizes=1
  Bias : Bias  Bias=1
  For Iterator : ForIterator  IterationLimit=nHistory-1
  Selector : Selector  InputPortWidth=nHistory  IndexOptions=Index vector (port)  Indices=[1 3]  OutputSizes=1
  Out1 : Outport
  wires:
  For Iterator/1 -> Bias/1, Selector/2
  Assignment/1 -> Out1/1
  In1/1 -> Assignment/1, Selector/1
  Bias/1 -> Assignment/3
  Selector/1 -> Assignment/2
